simulink model "Copy_of_Corneto_flight_program_control"  (R2021a)
settings: Solver=FixedStepAuto  StartTime=0.0  StopTime=inf  RelTol=1e-3
values from neighbouring files (symbols this model uses):
  den_lpf_d = den_lpf20    [Mainframe_init.m]    (also in load_autopilot.m)
  num_lpf_d = num_lpf20    [Mainframe_init.m]    (also in load_autopilot.m)
undefined symbols (not defined in the file or in its folder): Autopilot, AUX, dev, DiscIntNeverNeededParam, Flight_Logic, HIL_Data, Main, pwm_output0, pwm_output1, severity, text, x, y, z
libraries: simulink_extras x24, simulink x22, px4uORBlib x10, px4lib x10, px4Sensorslib x6, dspstat3 x2, sharedtransform x2
(part 2 of 3)

== system Copy_of_Corneto_flight_program_control/PixBlock2/Flight Logic/Subsystem4/Servo Commands2 ==
  Fin Cmd : Inport
  Recovery : Inport  Port=2
  Bus Selector : BusSelector  OutputSignals=signal1,signal2,signal3,signal4
  Cast To Double{1..5} (5 alike) : DataTypeConversion  OutDataTypeStr=uint16
  One4 : Constant  Value=0  OutDataTypeStr=boolean
  One5 : Constant  Value=2000  OutDataTypeStr=Inherit: Inherit via back propagation
  One6 : Constant  Value=1000  OutDataTypeStr=Inherit: Inherit via back propagation
  One7 : Constant  OutDataTypeStr=boolean
  PX4 PWM Output1 : px4lib/PX4 PWM Output  pwmDevice=Main (/dev/pwm_output0)  pwmChannel1_=on  pwmChannel2_=on  pwmChannel3_=on  pwmChannel4_=on  pwmChannel5_=on  pwmChannel6_=off  pwmChannel7_=off  pwmChannel8_=off  forceTerminateFailsafe=off  outputErrorStatus=off
      settings: SourceProductBaseCode=PX4AUTOPILOTS
  Switch : Switch  Criteria=u2 > Threshold
  Pwm : Outport
  wires:
  Bus Selector/4 -> Cast To Double1/1  "<signal4>"
  One4/1 -> PX4 PWM Output1/2
  Bus Selector/3 -> Cast To Double2/1  "<signal3>"
  Bus Selector/2 -> Cast To Double3/1  "<signal2>"
  Bus Selector/1 -> Cast To Double5/1  "<signal1>"
  Cast To Double4/1 -> PX4 PWM Output1/7
  Recovery/1 -> Switch/2
  One5/1 -> Switch/1
  One6/1 -> Switch/3
  Switch/1 -> Cast To Double4/1
  One7/1 -> PX4 PWM Output1/1
  Fin Cmd/1 -> Pwm/1, Bus Selector/1
  Cast To Double1/1 -> PX4 PWM Output1/6
  Cast To Double2/1 -> PX4 PWM Output1/5
  Cast To Double3/1 -> PX4 PWM Output1/4
  Cast To Double5/1 -> PX4 PWM Output1/3

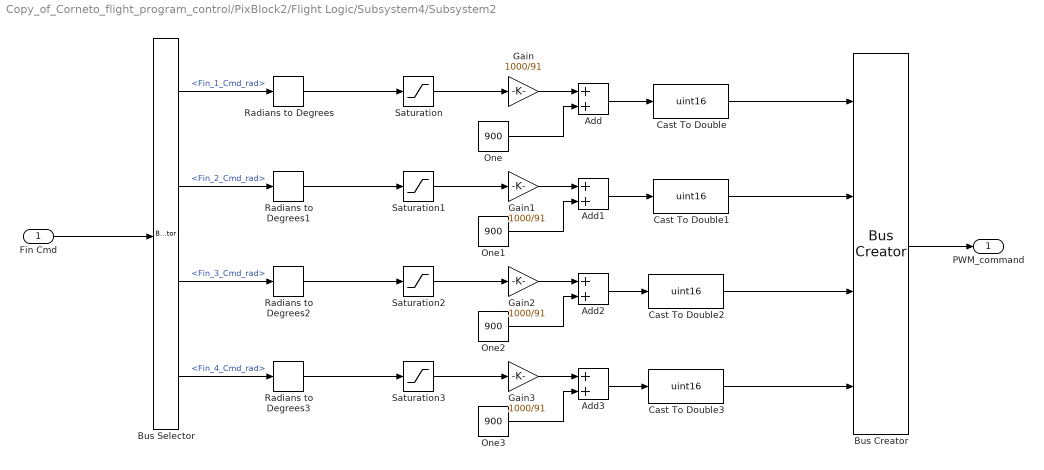
== system Copy_of_Corneto_flight_program_control/PixBlock2/Flight Logic/Subsystem4/Subsystem2 ==
  Fin Cmd : Inport
  Add{,1..3} (4 alike) : Sum
  Bus Selector : BusSelector  OutputSignals=Fin_1_Cmd_rad,Fin_2_Cmd_rad,Fin_3_Cmd_rad,Fin_4_Cmd_rad
  Bus Creator : BusCreator  Inputs=4
  Cast To Double{,1..3} (4 alike) : DataTypeConversion  OutDataTypeStr=uint16
  Gain{,1..3} (4 alike) : Gain  Gain=1000/91
  One{,1..3} (4 alike) : Constant  Value=900  OutDataTypeStr=Inherit: Inherit via back propagation
  Radians to Degrees{,1..3} (4 alike) : simulink_extras/Transformations/Radians to Degrees
  Saturation{,1..3} (4 alike) : Saturate  UpperLimit=20  LowerLimit=-20
  PWM_command : Outport
  wires:
  One2/1 -> Add2/2
  Add2/1 -> Cast To Double2/1
  Radians to Degrees2/1 -> Saturation2/1
  Cast To Double2/1 -> Bus Creator/3
  Gain/1 -> Add/1
  Bus Selector/1 -> Radians to Degrees/1  "<Fin_1_Cmd_rad>"
  Fin Cmd/1 -> Bus Selector/1
  Saturation/1 -> Gain/1
  Bus Selector/2 -> Radians to Degrees1/1  "<Fin_2_Cmd_rad>"
  Radians to Degrees/1 -> Saturation/1
  Saturation3/1 -> Gain3/1
  Cast To Double/1 -> Bus Creator/1
  Add3/1 -> Cast To Double3/1
  Gain1/1 -> Add1/1
  Saturation1/1 -> Gain1/1
  Radians to Degrees1/1 -> Saturation1/1
  Cast To Double3/1 -> Bus Creator/4
  Radians to Degrees3/1 -> Saturation3/1
  Gain2/1 -> Add2/1
  Cast To Double1/1 -> Bus Creator/2
  Bus Selector/3 -> Radians to Degrees2/1  "<Fin_3_Cmd_rad>"
  One1/1 -> Add1/2
  Bus Selector/4 -> Radians to Degrees3/1  "<Fin_4_Cmd_rad>"
  Add/1 -> Cast To Double/1
  One3/1 -> Add3/2
  Add1/1 -> Cast To Double1/1
  Gain3/1 -> Add3/1
  Saturation2/1 -> Gain2/1
  One/1 -> Add/2
  Bus Creator/1 -> PWM_command/1

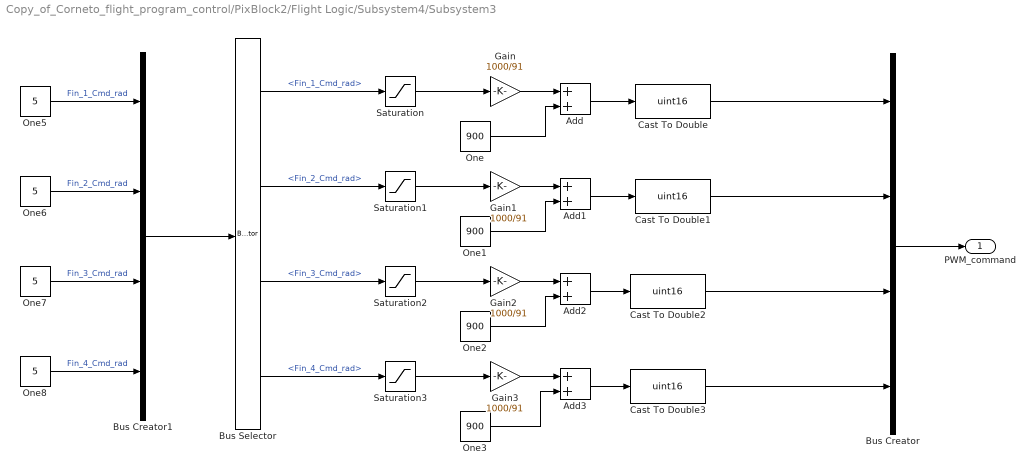
== system Copy_of_Corneto_flight_program_control/PixBlock2/Flight Logic/Subsystem4/Subsystem3 ==
  Add{,1..3} (4 alike) : Sum
  Bus Creator1 : BusCreator  Inputs=4
  Bus Selector : BusSelector  OutputSignals=Fin_1_Cmd_rad,Fin_2_Cmd_rad,Fin_3_Cmd_rad,Fin_4_Cmd_rad
  Bus Creator : BusCreator  Inputs=4
  Cast To Double{,1..3} (4 alike) : DataTypeConversion  OutDataTypeStr=uint16
  Gain{,1..3} (4 alike) : Gain  Gain=1000/91
  One{,1..3} (4 alike) : Constant  Value=900  OutDataTypeStr=Inherit: Inherit via back propagation
  One{5..8} (4 alike) : Constant  Value=5  OutDataTypeStr=Inherit: Inherit via back propagation
  Saturation{,1..3} (4 alike) : Saturate  UpperLimit=20  LowerLimit=-20
  PWM_command : Outport
  wires:
  One2/1 -> Add2/2
  Add2/1 -> Cast To Double2/1
  Cast To Double2/1 -> Bus Creator/3
  Gain/1 -> Add/1
  Bus Selector/1 -> Saturation/1  "<Fin_1_Cmd_rad>"
  Bus Creator1/1 -> Bus Selector/1
  Saturation/1 -> Gain/1
  Bus Selector/2 -> Saturation1/1  "<Fin_2_Cmd_rad>"
  Saturation3/1 -> Gain3/1
  Cast To Double/1 -> Bus Creator/1
  Add3/1 -> Cast To Double3/1
  Gain1/1 -> Add1/1
  Saturation1/1 -> Gain1/1
  Cast To Double3/1 -> Bus Creator/4
  Gain2/1 -> Add2/1
  Cast To Double1/1 -> Bus Creator/2
  Bus Selector/3 -> Saturation2/1  "<Fin_3_Cmd_rad>"
  One1/1 -> Add1/2
  Bus Selector/4 -> Saturation3/1  "<Fin_4_Cmd_rad>"
  Add/1 -> Cast To Double/1
  One3/1 -> Add3/2
  Add1/1 -> Cast To Double1/1
  Gain3/1 -> Add3/1
  Saturation2/1 -> Gain2/1
  One/1 -> Add/2
  Bus Creator/1 -> PWM_command/1
  One5/1 -> Bus Creator1/1  "Fin_1_Cmd_rad"
  One8/1 -> Bus Creator1/4  "Fin_4_Cmd_rad"
  One6/1 -> Bus Creator1/2  "Fin_2_Cmd_rad"
  One7/1 -> Bus Creator1/3  "Fin_3_Cmd_rad"

== system Copy_of_Corneto_flight_program_control/Subsystem/PixBlock2/Emulated Pixhawk/Autopilot ==
  Phi_cmd : Inport
  P_rms : Inport  Port=2
  Alt : Inport  Port=3
  Velocity : Inport  Port=4
  Phi : Inport  Port=5
  Reset_Integrators : Inport  Port=6
  Bus Creator3 : BusCreator  Inputs=3
  Discrete Transfer Fcn : DiscreteTransferFcn  Numerator=[num_lpf_d]  Denominator=[den_lpf_d]
  Phi_Control : Subsystem
  Zero : Constant  Value=0  OutDataTypeStr=Inherit: Inherit via back propagation
  Attitude_Commands : Outport  VectorParamsAs1DForOutWhenUnconnected=off
  P_filter : Outport  Port=2  VectorParamsAs1DForOutWhenUnconnected=off
  wires:
  P_rms/1 -> Discrete Transfer Fcn/1
  Velocity/1 -> Phi_Control/5(V_mps)
  Zero/1 -> [Delta_Cmd_Psi], [Delta_Cmd_Theta]
  [Delta_Cmd_Phi] -> Bus Creator3/1  "Phi_Cmd_rad"
  [Delta_Cmd_Theta] -> Bus Creator3/2  "Theta_Cmd_rad"
  Bus Creator3/1 -> Attitude_Commands/1
  [Delta_Cmd_Psi] -> Bus Creator3/3  "Psi_Cmd_rad"
  Alt/1 -> Phi_Control/6(h_m)
  Phi_Control/1(dela_cmd_rad) -> [Delta_Cmd_Phi]  "Phi_Cmd_rad"
  Discrete Transfer Fcn/1 -> P_filter/1, Phi_Control/3(p_rps)
  Phi/1 -> Phi_Control/2(phi_rad)
  Phi_cmd/1 -> Phi_Control/1(phi_cmd_rad)
  Reset_Integrators/1 -> Phi_Control/4(Reset Integrators)

== system Copy_of_Corneto_flight_program_control/Subsystem/PixBlock2/Emulated Pixhawk/Fin Allocation ==
  Attitude Cmd : Inport
  Bus Creator : BusCreator  Inputs=4
  Bus Selector : BusSelector  OutputSignals=Phi_Cmd_rad,Theta_Cmd_rad,Psi_Cmd_rad
  Demux : Demux
  Vector Concatenate1 : Concatenate  NumInputs=3
  control_allocation : Subsystem
  Fin Cmd : Outport  VectorParamsAs1DForOutWhenUnconnected=off
  wires:
  Demux/4 -> Bus Creator/4  "Fin_4_Cmd_rad"
  control_allocation/1(siB_cmd) -> Demux/1
  Bus Selector/3 -> Vector Concatenate1/3  "<Psi_Cmd_rad>"
  Vector Concatenate1/1 -> control_allocation/1(fin_cmd)  "fin_cmd"
  Bus Selector/1 -> Vector Concatenate1/1  "<Phi_Cmd_rad>"
  Demux/3 -> Bus Creator/3  "Fin_3_Cmd_rad"
  Bus Selector/2 -> Vector Concatenate1/2  "<Theta_Cmd_rad>"
  Demux/1 -> Bus Creator/1  "Fin_1_Cmd_rad"
  Bus Creator/1 -> Fin Cmd/1
  Attitude Cmd/1 -> Bus Selector/1
  Demux/2 -> Bus Creator/2  "Fin_2_Cmd_rad"

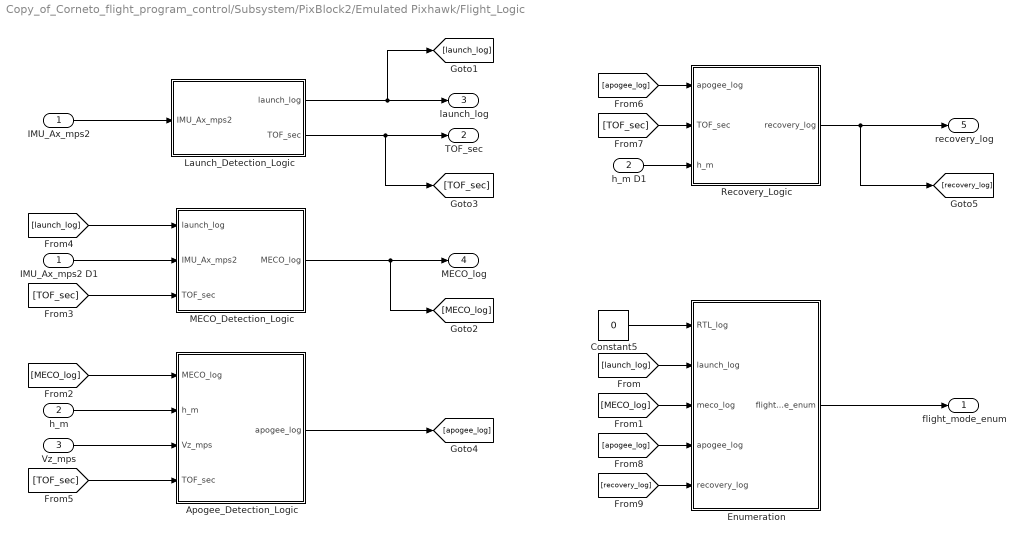
== system Copy_of_Corneto_flight_program_control/Subsystem/PixBlock2/Emulated Pixhawk/Flight_Logic ==
  IMU_Ax_mps2 : Inport
  h_m : Inport  Port=2
  Vz_mps : Inport  Port=3
  Apogee_Detection_Logic : Subsystem
  Constant5 : Constant  Value=0
  Enumeration : Subsystem
  IMU_Ax_mps2 D1 : InportShadow
  Launch_Detection_Logic : Subsystem
  MECO_Detection_Logic : Subsystem
  Recovery_Logic : Subsystem
  h_m D1 : InportShadow  Port=2
  flight_mode_enum : Outport
  TOF_sec : Outport  Port=2
  launch_log : Outport  Port=3
  MECO_log : Outport  Port=4
  recovery_log : Outport  Port=5
  wires:
  Enumeration/1(flight_mode_enum) -> flight_mode_enum/1
  [launch_log] -> Enumeration/2(launch_log)
  [MECO_log] -> Enumeration/3(meco_log)
  IMU_Ax_mps2/1 -> Launch_Detection_Logic/1(IMU_Ax_mps2)
  IMU_Ax_mps2 D1/1 -> MECO_Detection_Logic/2(IMU_Ax_mps2)
  Launch_Detection_Logic/1(launch_log) -> [launch_log], launch_log/1
  Launch_Detection_Logic/2(TOF_sec) -> [TOF_sec], TOF_sec/1
  [launch_log] -> MECO_Detection_Logic/1(launch_log)
  MECO_Detection_Logic/1(MECO_log) -> [MECO_log], MECO_log/1
  [MECO_log] -> Apogee_Detection_Logic/1(MECO_log)
  h_m/1 -> Apogee_Detection_Logic/2(h_m)
  Vz_mps/1 -> Apogee_Detection_Logic/3(Vz_mps)
  Apogee_Detection_Logic/1(apogee_log) -> [apogee_log]
  [TOF_sec] -> MECO_Detection_Logic/3(TOF_sec)
  [TOF_sec] -> Apogee_Detection_Logic/4(TOF_sec)
  Constant5/1 -> Enumeration/1(RTL_log)
  [apogee_log] -> Recovery_Logic/1(apogee_log)
  [TOF_sec] -> Recovery_Logic/2(TOF_sec)
  h_m D1/1 -> Recovery_Logic/3(h_m)
  Recovery_Logic/1(recovery_log) -> [recovery_log], recovery_log/1
  [apogee_log] -> Enumeration/4(apogee_log)
  [recovery_log] -> Enumeration/5(recovery_log)

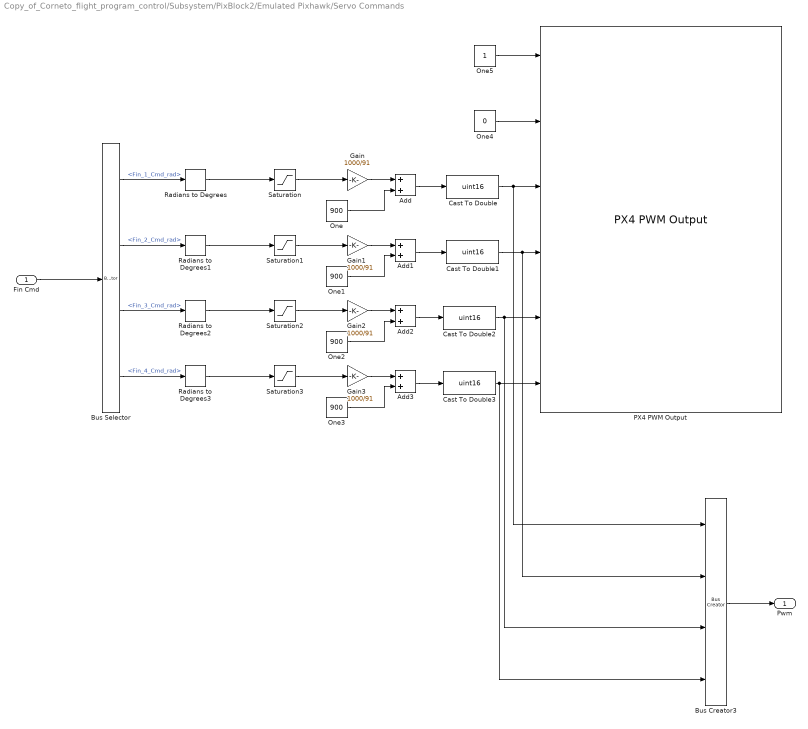
== system Copy_of_Corneto_flight_program_control/Subsystem/PixBlock2/Emulated Pixhawk/Servo Commands ==
  Fin Cmd : Inport
  Add{,1..3} (4 alike) : Sum
  Bus Creator3 : BusCreator  Inputs=4
  Bus Selector : BusSelector  OutputSignals=Fin_1_Cmd_rad,Fin_2_Cmd_rad,Fin_3_Cmd_rad,Fin_4_Cmd_rad
  Cast To Double{,1..3} (4 alike) : DataTypeConversion  OutDataTypeStr=uint16
  Gain{,1..3} (4 alike) : Gain  Gain=1000/91
  One{,1..3} (4 alike) : Constant  Value=900  OutDataTypeStr=Inherit: Inherit via back propagation
  One4 : Constant  Value=0  OutDataTypeStr=boolean  SampleTime=-1
  One5 : Constant  OutDataTypeStr=boolean  SampleTime=-1
  PX4 PWM Output : px4lib/PX4 PWM Output  pwmDevice=AUX (/dev/pwm_output1)  pwmChannel1_=on  pwmChannel2_=on  pwmChannel3_=on  pwmChannel4_=on  pwmChannel5_=off  pwmChannel6_=off  pwmChannel7_=off  pwmChannel8_=off  forceTerminateFailsafe=off  outputErrorStatus=off
      settings: SourceProductBaseCode=PX4AUTOPILOTS
  Radians to Degrees{,1..3} (4 alike) : simulink_extras/Transformations/Radians to Degrees
  Saturation{,1..3} (4 alike) : Saturate  UpperLimit=20  LowerLimit=-20
  Pwm : Outport
  wires:
  Saturation2/1 -> Gain2/1
  One4/1 -> PX4 PWM Output/2
  One/1 -> Add/2
  One2/1 -> Add2/2
  Add1/1 -> Cast To Double1/1
  Gain2/1 -> Add2/1
  Radians to Degrees1/1 -> Saturation1/1
  Add2/1 -> Cast To Double2/1
  Fin Cmd/1 -> Bus Selector/1
  Bus Selector/2 -> Radians to Degrees1/1  "<Fin_2_Cmd_rad>"
  Gain/1 -> Add/1
  Bus Selector/4 -> Radians to Degrees3/1  "<Fin_4_Cmd_rad>"
  One3/1 -> Add3/2
  Saturation/1 -> Gain/1
  Gain1/1 -> Add1/1
  Saturation3/1 -> Gain3/1
  Gain3/1 -> Add3/1
  Radians to Degrees3/1 -> Saturation3/1
  Bus Selector/1 -> Radians to Degrees/1  "<Fin_1_Cmd_rad>"
  Bus Selector/3 -> Radians to Degrees2/1  "<Fin_3_Cmd_rad>"
  Saturation1/1 -> Gain1/1
  Add3/1 -> Cast To Double3/1
  Radians to Degrees2/1 -> Saturation2/1
  Radians to Degrees/1 -> Saturation/1
  One1/1 -> Add1/2
  Add/1 -> Cast To Double/1
  Bus Creator3/1 -> Pwm/1
  Cast To Double/1 -> PX4 PWM Output/3, Bus Creator3/1
  Cast To Double1/1 -> PX4 PWM Output/4, Bus Creator3/2
  Cast To Double2/1 -> PX4 PWM Output/5, Bus Creator3/3
  Cast To Double3/1 -> PX4 PWM Output/6, Bus Creator3/4
  One5/1 -> PX4 PWM Output/1

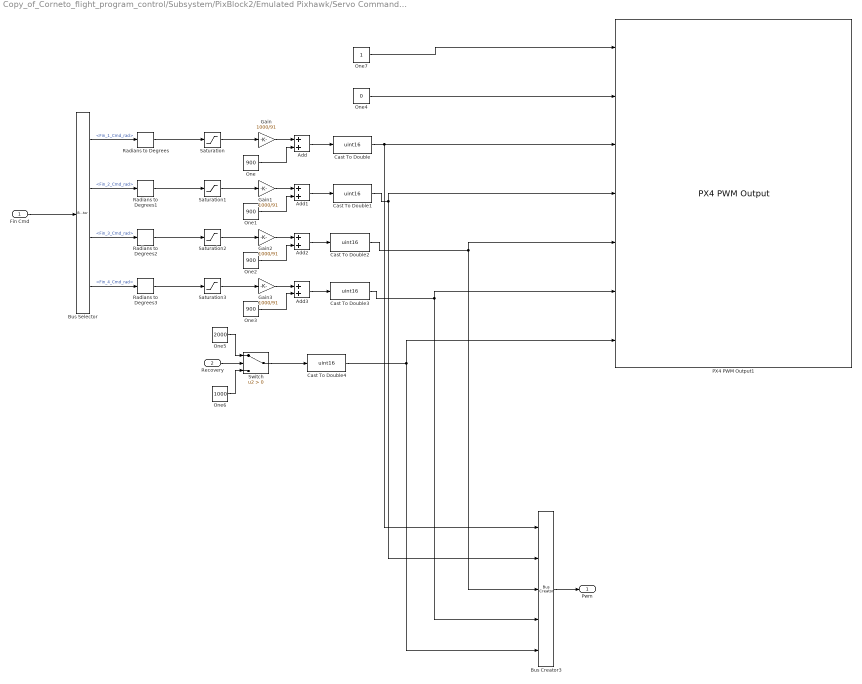
== system Copy_of_Corneto_flight_program_control/Subsystem/PixBlock2/Emulated Pixhawk/Servo Commands1 ==
  Fin Cmd : Inport
  Recovery : Inport  Port=2
  Add{,1..3} (4 alike) : Sum
  Bus Creator3 : BusCreator  Inputs=5
  Bus Selector : BusSelector  OutputSignals=Fin_1_Cmd_rad,Fin_2_Cmd_rad,Fin_3_Cmd_rad,Fin_4_Cmd_rad
  Cast To Double{,1..4} (5 alike) : DataTypeConversion  OutDataTypeStr=uint16
  Gain{,1..3} (4 alike) : Gain  Gain=1000/91
  One{,1..3} (4 alike) : Constant  Value=900  OutDataTypeStr=Inherit: Inherit via back propagation
  One4 : Constant  Value=0  OutDataTypeStr=boolean
  One5 : Constant  Value=2000  OutDataTypeStr=Inherit: Inherit via back propagation
  One6 : Constant  Value=1000  OutDataTypeStr=Inherit: Inherit via back propagation
  One7 : Constant  OutDataTypeStr=boolean
  PX4 PWM Output1 : px4lib/PX4 PWM Output  pwmDevice=Main (/dev/pwm_output0)  pwmChannel1_=on  pwmChannel2_=on  pwmChannel3_=on  pwmChannel4_=on  pwmChannel5_=on  pwmChannel6_=off  pwmChannel7_=off  pwmChannel8_=off  forceTerminateFailsafe=off  outputErrorStatus=off
      settings: SourceProductBaseCode=PX4AUTOPILOTS
  Radians to Degrees{,1..3} (4 alike) : simulink_extras/Transformations/Radians to Degrees
  Saturation{,1..3} (4 alike) : Saturate  UpperLimit=20  LowerLimit=-20
  Switch : Switch  Criteria=u2 > Threshold
  Pwm : Outport
  wires:
  Saturation2/1 -> Gain2/1
  Cast To Double3/1 -> Bus Creator3/4, PX4 PWM Output1/6
  One4/1 -> PX4 PWM Output1/2
  One/1 -> Add/2
  One2/1 -> Add2/2
  Add1/1 -> Cast To Double1/1
  Gain2/1 -> Add2/1
  Radians to Degrees1/1 -> Saturation1/1
  Cast To Double2/1 -> Bus Creator3/3, PX4 PWM Output1/5
  Add2/1 -> Cast To Double2/1
  Fin Cmd/1 -> Bus Selector/1
  Cast To Double1/1 -> Bus Creator3/2, PX4 PWM Output1/4
  Bus Selector/2 -> Radians to Degrees1/1  "<Fin_2_Cmd_rad>"
  Gain/1 -> Add/1
  Bus Selector/4 -> Radians to Degrees3/1  "<Fin_4_Cmd_rad>"
  One3/1 -> Add3/2
  Saturation/1 -> Gain/1
  Gain1/1 -> Add1/1
  Saturation3/1 -> Gain3/1
  Gain3/1 -> Add3/1
  Radians to Degrees3/1 -> Saturation3/1
  Bus Selector/1 -> Radians to Degrees/1  "<Fin_1_Cmd_rad>"
  Bus Selector/3 -> Radians to Degrees2/1  "<Fin_3_Cmd_rad>"
  Saturation1/1 -> Gain1/1
  Cast To Double/1 -> Bus Creator3/1, PX4 PWM Output1/3
  Add3/1 -> Cast To Double3/1
  Radians to Degrees2/1 -> Saturation2/1
  Radians to Degrees/1 -> Saturation/1
  One1/1 -> Add1/2
  Add/1 -> Cast To Double/1
  Cast To Double4/1 -> Bus Creator3/5, PX4 PWM Output1/7
  Recovery/1 -> Switch/2
  One5/1 -> Switch/1
  One6/1 -> Switch/3
  Switch/1 -> Cast To Double4/1
  One7/1 -> PX4 PWM Output1/1
  Bus Creator3/1 -> Pwm/1

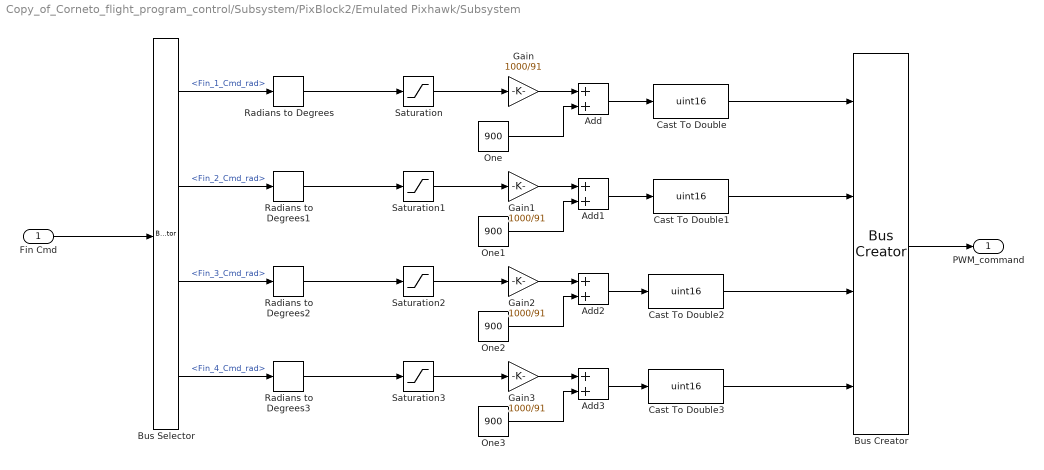
== system Copy_of_Corneto_flight_program_control/Subsystem/PixBlock2/Emulated Pixhawk/Subsystem ==
  Fin Cmd : Inport
  Add{,1..3} (4 alike) : Sum
  Bus Selector : BusSelector  OutputSignals=Fin_1_Cmd_rad,Fin_2_Cmd_rad,Fin_3_Cmd_rad,Fin_4_Cmd_rad
  Bus Creator : BusCreator  Inputs=4
  Cast To Double{,1..3} (4 alike) : DataTypeConversion  OutDataTypeStr=uint16
  Gain{,1..3} (4 alike) : Gain  Gain=1000/91
  One{,1..3} (4 alike) : Constant  Value=900  OutDataTypeStr=Inherit: Inherit via back propagation
  Radians to Degrees{,1..3} (4 alike) : simulink_extras/Transformations/Radians to Degrees
  Saturation{,1..3} (4 alike) : Saturate  UpperLimit=20  LowerLimit=-20
  PWM_command : Outport
  wires:
  One2/1 -> Add2/2
  Add2/1 -> Cast To Double2/1
  Radians to Degrees2/1 -> Saturation2/1
  Cast To Double2/1 -> Bus Creator/3
  Gain/1 -> Add/1
  Bus Selector/1 -> Radians to Degrees/1  "<Fin_1_Cmd_rad>"
  Fin Cmd/1 -> Bus Selector/1
  Saturation/1 -> Gain/1
  Bus Selector/2 -> Radians to Degrees1/1  "<Fin_2_Cmd_rad>"
  Radians to Degrees/1 -> Saturation/1
  Saturation3/1 -> Gain3/1
  Cast To Double/1 -> Bus Creator/1
  Add3/1 -> Cast To Double3/1
  Gain1/1 -> Add1/1
  Saturation1/1 -> Gain1/1
  Radians to Degrees1/1 -> Saturation1/1
  Cast To Double3/1 -> Bus Creator/4
  Radians to Degrees3/1 -> Saturation3/1
  Gain2/1 -> Add2/1
  Cast To Double1/1 -> Bus Creator/2
  Bus Selector/3 -> Radians to Degrees2/1  "<Fin_3_Cmd_rad>"
  One1/1 -> Add1/2
  Bus Selector/4 -> Radians to Degrees3/1  "<Fin_4_Cmd_rad>"
  Add/1 -> Cast To Double/1
  One3/1 -> Add3/2
  Add1/1 -> Cast To Double1/1
  Gain3/1 -> Add3/1
  Saturation2/1 -> Gain2/1
  One/1 -> Add/2
  Bus Creator/1 -> PWM_command/1

== system Copy_of_Corneto_flight_program_control/Subsystem/PixBlock2/Emulated Pixhawk/Subsystem1 ==
  Add{,1..3} (4 alike) : Sum
  Bus Creator1 : BusCreator  Inputs=4
  Bus Selector : BusSelector  OutputSignals=Fin_1_Cmd_rad,Fin_2_Cmd_rad,Fin_3_Cmd_rad,Fin_4_Cmd_rad
  Bus Creator : BusCreator  Inputs=4
  Cast To Double{,1..3} (4 alike) : DataTypeConversion  OutDataTypeStr=uint16
  Gain{,1..3} (4 alike) : Gain  Gain=1000/91
  One{,1..3} (4 alike) : Constant  Value=900  OutDataTypeStr=Inherit: Inherit via back propagation
  One{5..8} (4 alike) : Constant  Value=5  OutDataTypeStr=Inherit: Inherit via back propagation
  Saturation{,1..3} (4 alike) : Saturate  UpperLimit=20  LowerLimit=-20
  PWM_command : Outport
  wires:
  One2/1 -> Add2/2
  Add2/1 -> Cast To Double2/1
  Cast To Double2/1 -> Bus Creator/3
  Gain/1 -> Add/1
  Bus Selector/1 -> Saturation/1  "<Fin_1_Cmd_rad>"
  Bus Creator1/1 -> Bus Selector/1
  Saturation/1 -> Gain/1
  Bus Selector/2 -> Saturation1/1  "<Fin_2_Cmd_rad>"
  Saturation3/1 -> Gain3/1
  Cast To Double/1 -> Bus Creator/1
  Add3/1 -> Cast To Double3/1
  Gain1/1 -> Add1/1
  Saturation1/1 -> Gain1/1
  Cast To Double3/1 -> Bus Creator/4
  Gain2/1 -> Add2/1
  Cast To Double1/1 -> Bus Creator/2
  Bus Selector/3 -> Saturation2/1  "<Fin_3_Cmd_rad>"
  One1/1 -> Add1/2
  Bus Selector/4 -> Saturation3/1  "<Fin_4_Cmd_rad>"
  Add/1 -> Cast To Double/1
  One3/1 -> Add3/2
  Add1/1 -> Cast To Double1/1
  Gain3/1 -> Add3/1
  Saturation2/1 -> Gain2/1
  One/1 -> Add/2
  Bus Creator/1 -> PWM_command/1
  One5/1 -> Bus Creator1/1  "Fin_1_Cmd_rad"
  One8/1 -> Bus Creator1/4  "Fin_4_Cmd_rad"
  One6/1 -> Bus Creator1/2  "Fin_2_Cmd_rad"
  One7/1 -> Bus Creator1/3  "Fin_3_Cmd_rad"

== system Copy_of_Corneto_flight_program_control/PixBlock2/Flight Logic/Autopilot/Phi_Control/Gain_Lookup ==
  V_mps : Inport
  h_m : Inport  Port=2
  1-D Lookup Table1 : Lookup_n-D  BreakpointsForDimension1=Autopilot.Ay.h_bkpts_m  BreakpointsForDimension2=Autopilot.Ay.V_bkpts_mps  Table=Autopilot.Ay.Kp_r_vec  ExtrapMethod=Clip  UseLastTableValue=on  InternalRulePriority=Speed  RndMeth=Simplest  InputSameDT=on
      settings: InputPortMap=u0,u1
      settings: AttributesFormatString=|
      | %<Table>
      | %<BreakpointsForDimension1>
      | %<BreakpointsForDimension2>
  1-D Lookup Table2 : Lookup_n-D  BreakpointsForDimension1=Autopilot.Ay.h_bkpts_m  BreakpointsForDimension2=Autopilot.Ay.V_bkpts_mps  Table=Autopilot.Ay.Kp_ay_vec  ExtrapMethod=Clip  UseLastTableValue=on  InternalRulePriority=Speed  RndMeth=Simplest  InputSameDT=on
      settings: InputPortMap=u0,u1
      settings: AttributesFormatString=|
      | %<Table>
      | %<BreakpointsForDimension1>
      | %<BreakpointsForDimension2>
  1-D Lookup Table3 : Lookup_n-D  BreakpointsForDimension1=Autopilot.Phi.h_bkpts_m  BreakpointsForDimension2=Autopilot.Phi.V_bkpts_mps  Table=Autopilot.Phi.Kp_p_vec  ExtrapMethod=Clip  UseLastTableValue=on  InternalRulePriority=Speed  RndMeth=Simplest  InputSameDT=on
      settings: InputPortMap=u0,u1
      settings: AttributesFormatString=|
      | %<Table>
      | %<BreakpointsForDimension1>
      | %<BreakpointsForDimension2>
  1-D Lookup Table4 : Lookup_n-D  BreakpointsForDimension1=Autopilot.Phi.h_bkpts_m  BreakpointsForDimension2=Autopilot.Phi.V_bkpts_mps  Table=Autopilot.Phi.Ki_phi_vec  ExtrapMethod=Clip  UseLastTableValue=on  InternalRulePriority=Speed  RndMeth=Simplest  InputSameDT=on
      settings: InputPortMap=u0,u1
      settings: AttributesFormatString=|
      | %<Table>
      | %<BreakpointsForDimension1>
      | %<BreakpointsForDimension2>
  1-D Lookup Table5 : Lookup_n-D  BreakpointsForDimension1=Autopilot.Phi.h_bkpts_m  BreakpointsForDimension2=Autopilot.Phi.V_bkpts_mps  Table=Autopilot.Phi.Kp_phi_vec  ExtrapMethod=Clip  UseLastTableValue=on  InternalRulePriority=Speed  RndMeth=Simplest  InputSameDT=on
      settings: InputPortMap=u0,u1
      settings: AttributesFormatString=|
      | %<Table>
      | %<BreakpointsForDimension1>
      | %<BreakpointsForDimension2>
  1-D Lookup Table6 : Lookup_n-D  BreakpointsForDimension1=Autopilot.Ay.h_bkpts_m  BreakpointsForDimension2=Autopilot.Ay.V_bkpts_mps  Table=Autopilot.Ay.Ki_ay_vec  ExtrapMethod=Clip  UseLastTableValue=on  InternalRulePriority=Speed  RndMeth=Simplest  InputSameDT=on
      settings: InputPortMap=u0,u1
      settings: AttributesFormatString=|
      | %<Table>
      | %<BreakpointsForDimension1>
      | %<BreakpointsForDimension2>
  Bus Creator1 : BusCreator  Inputs=6
  V_mps D{1..5} (5 alike) : InportShadow
  h_m D{1..5} (5 alike) : InportShadow  Port=2
  Gains : Outport
  wires:
  h_m/1 -> 1-D Lookup Table3/1
  Bus Creator1/1 -> Gains/1
  1-D Lookup Table5/1 -> Bus Creator1/3  "Kp_phi"
  1-D Lookup Table4/1 -> Bus Creator1/2  "Ki_phi"
  1-D Lookup Table3/1 -> Bus Creator1/1  "Kp_p"
  V_mps/1 -> 1-D Lookup Table3/2
  h_m D1/1 -> 1-D Lookup Table4/1
  V_mps D1/1 -> 1-D Lookup Table4/2
  h_m D2/1 -> 1-D Lookup Table5/1
  V_mps D2/1 -> 1-D Lookup Table5/2
  1-D Lookup Table2/1 -> Bus Creator1/6  "Kp_ay"
  1-D Lookup Table6/1 -> Bus Creator1/5  "Ki_ay"
  1-D Lookup Table1/1 -> Bus Creator1/4  "Kp_r"
  h_m D3/1 -> 1-D Lookup Table1/1
  V_mps D3/1 -> 1-D Lookup Table1/2
  h_m D4/1 -> 1-D Lookup Table6/1
  V_mps D4/1 -> 1-D Lookup Table6/2
  h_m D5/1 -> 1-D Lookup Table2/1
  V_mps D5/1 -> 1-D Lookup Table2/2

== system Copy_of_Corneto_flight_program_control/PixBlock2/Flight Logic/Flight_Logic/Apogee_Detection_Logic/Enable_Timer_Logic ==
  enable_timer : Inport
  Constant : Constant
  Constant1 : Constant  Value=0
  Discrete-Time Integrator : DiscreteIntegrator  ExternalReset=level  InitialConditionSource=external  SampleTime=-1  ICPrevOutput=DiscIntNeverNeededParam  ICPrevScaledInput=DiscIntNeverNeededParam
  NOT : Logic  Operator=NOT  AllPortsSameDT=off  OutDataTypeStr=boolean
  timer : Outport
  wires:
  NOT/1 -> Discrete-Time Integrator/2
  Discrete-Time Integrator/1 -> timer/1  "apogee_detect_timer_sec"
  Constant1/1 -> Discrete-Time Integrator/3
  Constant/1 -> Discrete-Time Integrator/1
  enable_timer/1 -> NOT/1  "enable_timer"

== system Copy_of_Corneto_flight_program_control/PixBlock2/Flight Logic/Flight_Logic/Apogee_Detection_Logic/Latch_Signal ==
  signal : Inport
  Memory : Memory  InheritSampleTime=on
  Switch1 : Switch  Criteria=u2 ~= 0
      settings: AttributesFormatString=%<Criteria>
  signal_latched : Outport
  wires:
  signal/1 -> Switch1/2, Switch1/1
  Switch1/1 -> Memory/1, signal_latched/1
  Memory/1 -> Switch1/3

== system Copy_of_Corneto_flight_program_control/PixBlock2/Flight Logic/Flight_Logic/Launch_Detection_Logic/Enable_Timer_Logic ==
  accel_threshold_log : Inport
  launch_latched : Inport  Port=2
  AND : Logic  Operator=OR  AllPortsSameDT=off  OutDataTypeStr=boolean
  Constant : Constant
  Constant1 : Constant  Value=0
  Discrete-Time Integrator : DiscreteIntegrator  ExternalReset=level  InitialConditionSource=external  SampleTime=-1  ICPrevOutput=DiscIntNeverNeededParam  ICPrevScaledInput=DiscIntNeverNeededParam
  NOT : Logic  Operator=NOT  AllPortsSameDT=off  OutDataTypeStr=boolean
  time_since_launch : Outport
  wires:
  launch_latched/1 -> AND/2
  AND/1 -> NOT/1  "enable_timer"
  Constant/1 -> Discrete-Time Integrator/1
  Constant1/1 -> Discrete-Time Integrator/3
  Discrete-Time Integrator/1 -> time_since_launch/1  "launch_detect_timer_sec"
  accel_threshold_log/1 -> AND/1
  NOT/1 -> Discrete-Time Integrator/2

== system Copy_of_Corneto_flight_program_control/PixBlock2/Flight Logic/Flight_Logic/Launch_Detection_Logic/Latch_Signal ==
  signal : Inport
  Memory : Memory  InheritSampleTime=on  LinearizeAsDelay=on
  Switch1 : Switch  Criteria=u2 ~= 0
      settings: AttributesFormatString=%<Criteria>
  signal_latched : Outport
  wires:
  Memory/1 -> Switch1/3
  Switch1/1 -> signal_latched/1, Memory/1
  signal/1 -> Switch1/1, Switch1/2

== system Copy_of_Corneto_flight_program_control/PixBlock2/Flight Logic/Flight_Logic/MECO_Detection_Logic/Enable_Timer_Logic ==
  enable_timer : Inport
  Constant : Constant
  Constant1 : Constant  Value=0
  Discrete-Time Integrator : DiscreteIntegrator  ExternalReset=level  InitialConditionSource=external  SampleTime=-1  ICPrevOutput=DiscIntNeverNeededParam  ICPrevScaledInput=DiscIntNeverNeededParam
  NOT : Logic  Operator=NOT  AllPortsSameDT=off  OutDataTypeStr=boolean
  timer : Outport
  wires:
  enable_timer/1 -> NOT/1  "enable_timer"
  Constant/1 -> Discrete-Time Integrator/1
  Constant1/1 -> Discrete-Time Integrator/3
  Discrete-Time Integrator/1 -> timer/1  "MECO_detect_timer_sec"
  NOT/1 -> Discrete-Time Integrator/2

== system Copy_of_Corneto_flight_program_control/PixBlock2/Flight Logic/Flight_Logic/MECO_Detection_Logic/Latch_Signal ==
  signal : Inport
  Memory : Memory  InheritSampleTime=on
  Switch1 : Switch  Criteria=u2 ~= 0
      settings: AttributesFormatString=%<Criteria>
  signal_latched : Outport
  wires:
  Memory/1 -> Switch1/3
  Switch1/1 -> signal_latched/1, Memory/1
  signal/1 -> Switch1/1, Switch1/2

== system Copy_of_Corneto_flight_program_control/PixBlock2/Flight Logic/Flight_Logic/Recovery_Logic/Enable_Timer_Logic ==
  enable_timer : Inport
  Constant : Constant
  Constant1 : Constant  Value=0
  Discrete-Time Integrator : DiscreteIntegrator  ExternalReset=level  InitialConditionSource=external  SampleTime=-1  ICPrevOutput=DiscIntNeverNeededParam  ICPrevScaledInput=DiscIntNeverNeededParam
  NOT : Logic  Operator=NOT  AllPortsSameDT=off  OutDataTypeStr=boolean
  timer : Outport
  wires:
  NOT/1 -> Discrete-Time Integrator/2
  Discrete-Time Integrator/1 -> timer/1  "recovery_detect_timer_sec"
  Constant1/1 -> Discrete-Time Integrator/3
  Constant/1 -> Discrete-Time Integrator/1
  enable_timer/1 -> NOT/1  "enable_timer"

== system Copy_of_Corneto_flight_program_control/PixBlock2/Flight Logic/Flight_Logic/Recovery_Logic/Latch_Signal ==
  signal : Inport
  Memory : Memory  InheritSampleTime=on
  Switch1 : Switch  Criteria=u2 ~= 0
      settings: AttributesFormatString=%<Criteria>
  signal_latched : Outport
  wires:
  signal/1 -> Switch1/2, Switch1/1
  Switch1/1 -> Memory/1, signal_latched/1
  Memory/1 -> Switch1/3

== system Copy_of_Corneto_flight_program_control/Subsystem/PixBlock2/Emulated Pixhawk/Autopilot/Phi_Control ==
  phi_cmd_rad : Inport
  phi_rad : Inport  Port=2
  p_rps : Inport  Port=3
  Reset Integrators : Inport  Port=4
  V_mps : Inport  Port=5
  h_m : Inport  Port=6
  Bus Selector : BusSelector  OutputSignals=Kp_p,Ki_phi,Kp_phi,Kp_r,Ki_ay,Kp_ay
  Constant : Constant  Value=0  OutDataTypeStr=single  SampleTime=-1
  Discrete-Time Integrator : DiscreteIntegrator  ExternalReset=level  InitialConditionSource=external  SampleTime=-1  OutDataTypeStr=single  ICPrevOutput=DiscIntNeverNeededParam  ICPrevScaledInput=DiscIntNeverNeededParam
  Gain_Lookup : Subsystem
  Product1 : Product
  Product2 : Product
  Product3 : Product
  Sum3 : Sum  Inputs=|+-
  Sum4 : Sum  Inputs=++|
  Sum5 : Sum  Inputs=|+-
  dela_cmd_rad : Outport
  wires:
  phi_cmd_rad/1 -> Sum3/1
  Reset Integrators/1 -> Discrete-Time Integrator/2
  p_rps/1 -> Sum5/2
  phi_rad/1 -> Sum3/2
  Product2/1 -> Sum4/1
  Sum3/1 -> Product3/2, Product2/2
  Constant/1 -> Discrete-Time Integrator/3
  Sum5/1 -> Product1/2
  [Ki_phi] -> Product3/1
  Product1/1 -> dela_cmd_rad/1
  [Kp_p] -> Product1/1
  [Kp_phi] -> Product2/1
  Discrete-Time Integrator/1 -> Sum4/2  "phi_int"
  Sum4/1 -> Sum5/1
  Product3/1 -> Discrete-Time Integrator/1
  h_m/1 -> Gain_Lookup/2(h_m)
  Bus Selector/6 -> [Kp_ay]  "<Kp_ay>"
  Bus Selector/5 -> [Ki_ay]  "<Ki_ay>"
  Bus Selector/2 -> [Ki_phi]  "<Ki_phi>"
  Bus Selector/1 -> [Kp_p]  "<Kp_p>"
  V_mps/1 -> Gain_Lookup/1(V_mps)
  Bus Selector/4 -> [Kp_r]  "<Kp_r>"
  Gain_Lookup/1(Gains) -> Bus Selector/1
  Bus Selector/3 -> [Kp_phi]  "<Kp_phi>"

== system Copy_of_Corneto_flight_program_control/Subsystem/PixBlock2/Emulated Pixhawk/Fin Allocation/control_allocation ==
  fin_cmd : Inport
  Constant7 : Constant  Value=HIL_Data.FDM.Tr4r3  OutDataTypeStr=single
  Product : Product  Multiplication=Matrix(*)
  siB_cmd : Outport  VectorParamsAs1DForOutWhenUnconnected=off
  wires:
  Constant7/1 -> Product/1
  fin_cmd/1 -> Product/2
  Product/1 -> siB_cmd/1  "siB_cmd"

== system Copy_of_Corneto_flight_program_control/Subsystem/PixBlock2/Emulated Pixhawk/Flight_Logic/Apogee_Detection_Logic ==
  MECO_log : Inport
  h_m : Inport  Port=2
  Vz_mps : Inport  Port=3
  TOF_sec : Inport  Port=4
  AND : Logic  Inputs=3  AllPortsSameDT=off  OutDataTypeStr=boolean
  AND1 : Logic  Operator=OR  AllPortsSameDT=off  OutDataTypeStr=boolean
  Compare To Constant : simulink/Logic and Bit Operations/Compare To Constant  relop=>  const=0  OutDataTypeStr=boolean
  Compare To Constant1 : simulink/Logic and Bit Operations/Compare To Constant  relop=>=  const=Flight_Logic.h_apogee_timer_threshold_sec  OutDataTypeStr=boolean
      settings: AttributesFormatString=|
      | %<relop>
      | %<const>
  Compare To Constant3 : simulink/Logic and Bit Operations/Compare To Constant  relop=>=  const=Flight_Logic.apogee_timeout_TOF_sec  OutDataTypeStr=boolean
      settings: AttributesFormatString=|
      | %<relop>
      | %<const>
  Detect Decrease : simulink/Logic and Bit Operations/Detect Decrease  vinit=0.0  OutDataTypeStr=uint8
  Enable_Timer_Logic : Subsystem
  Latch_Signal : Subsystem
  Moving Average1 : dspstat3/Moving Average  Method=Sliding window  ForgettingFactorPort=off  SpecifyWindowLength=on  WindowLength=guidc_n_window  ForgettingFactor=0.9  SimulateUsing=Code generation
  apogee_log : Outport
  wires:
  AND1/1 -> apogee_log/1  "apogee_log"
  AND/1 -> Latch_Signal/1(signal)
  h_m/1 -> Moving Average1/1
  MECO_log/1 -> AND/1
  Moving Average1/1 -> Detect Decrease/1  "hBE_mf"
  Detect Decrease/1 -> Enable_Timer_Logic/1(enable_timer)  "flag_I_hBE"
  Enable_Timer_Logic/1(timer) -> Compare To Constant1/1
  Compare To Constant1/1 -> AND/2  "apogee_timer_log"
  Vz_mps/1 -> Compare To Constant/1
  Compare To Constant/1 -> AND/3  "apogee_vz_log"
  Latch_Signal/1(signal_latched) -> AND1/1  "apogee_latched"
  TOF_sec/1 -> Compare To Constant3/1
  Compare To Constant3/1 -> AND1/2  "apogee_timeout_log"

== system Copy_of_Corneto_flight_program_control/Subsystem/PixBlock2/Emulated Pixhawk/Flight_Logic/Enumeration ==
  RTL_log : Inport
  launch_log : Inport  Port=2
  meco_log : Inport  Port=3
  apogee_log : Inport  Port=4
  recovery_log : Inport  Port=5
  Constant : Constant
  Constant1 : Constant  Value=200
  Constant2 : Constant  Value=300
  Constant3 : Constant  Value=400
  Constant4 : Constant  Value=600
  Constant5 : Constant  Value=0
  Constant6 : Constant  Value=500
  Switch{,1..4} (5 alike) : Switch  Criteria=u2 ~= 0
  Terminator : Terminator
  flight_mode_enum : Outport
  wires:
  Switch/1 -> Switch1/3
  Constant3/1 -> Switch2/1
  Constant4/1 -> Switch3/1
  RTL_log/1 -> Switch/2
  Constant1/1 -> Switch/1
  Constant/1 -> Switch/3
  Switch3/1 -> flight_mode_enum/1  "flight_mode_enum"
  meco_log/1 -> Switch2/2
  launch_log/1 -> Switch1/2
  Constant2/1 -> Switch1/1
  Switch2/1 -> Switch4/3
  Switch1/1 -> Switch2/3
  Constant5/1 -> Switch4/2
  Constant6/1 -> Switch4/1
  Switch4/1 -> Switch3/3
  recovery_log/1 -> Switch3/2
  apogee_log/1 -> Terminator/1

== system Copy_of_Corneto_flight_program_control/Subsystem/PixBlock2/Emulated Pixhawk/Flight_Logic/Launch_Detection_Logic ==
  IMU_Ax_mps2 : Inport
  AND : Logic  AllPortsSameDT=off  OutDataTypeStr=boolean
  Compare To Constant : simulink/Logic and Bit Operations/Compare To Constant  relop=>=  const=Flight_Logic.Ax_launch_accel_threshold_mps2  OutDataTypeStr=boolean
      settings: AttributesFormatString=|
      | %<relop>
      | %<const>
  Compare To Constant1 : simulink/Logic and Bit Operations/Compare To Constant  relop=>=  const=Flight_Logic.Ax_launch_timer_threshold_sec  OutDataTypeStr=boolean
      settings: AttributesFormatString=|
      | %<relop>
      | %<const>
  Constant : Constant  Value=0
  Enable_Timer_Logic : Subsystem
  Latch_Signal : Subsystem
  Memory : Memory  InheritSampleTime=on  LinearizeAsDelay=on
  Switch : Switch  Criteria=u2 ~= 0
  launch_log : Outport
  TOF_sec : Outport  Port=2
  wires:
  Compare To Constant/1 -> AND/1, Enable_Timer_Logic/1(accel_threshold_log)  "launch_Ax_log"
  Enable_Timer_Logic/1(time_since_launch) -> Switch/1, Compare To Constant1/1
  Compare To Constant1/1 -> AND/2  "launch_timer_log"
  AND/1 -> Latch_Signal/1(signal)
  IMU_Ax_mps2/1 -> Compare To Constant/1
  Latch_Signal/1(signal_latched) -> [launch_latched], launch_log/1  "launch_log"
  [launch_latched] -> Memory/1
  Memory/1 -> Enable_Timer_Logic/2(launch_latched)
  [launch_latched] -> Switch/2
  Switch/1 -> TOF_sec/1  "TOF_sec"
  Constant/1 -> Switch/3

== system Copy_of_Corneto_flight_program_control/Subsystem/PixBlock2/Emulated Pixhawk/Flight_Logic/MECO_Detection_Logic ==
  launch_log : Inport
  IMU_Ax_mps2 : Inport  Port=2
  TOF_sec : Inport  Port=3
  AND : Logic  AllPortsSameDT=off  OutDataTypeStr=boolean
  AND1 : Logic  Operator=OR  AllPortsSameDT=off  OutDataTypeStr=boolean
  Compare To Constant1 : simulink/Logic and Bit Operations/Compare To Constant  relop=>=  const=Flight_Logic.Ax_MECO_timer_threshold_sec  OutDataTypeStr=boolean
      settings: AttributesFormatString=|
      | %<relop>
      | %<const>
  Compare To Constant2 : simulink/Logic and Bit Operations/Compare To Constant  relop=<=  const=0  OutDataTypeStr=boolean
      settings: AttributesFormatString=|
      | %<relop>
      | %<const>
  Compare To Constant3 : simulink/Logic and Bit Operations/Compare To Constant  relop=>=  const=Flight_Logic.MECO_timeout_TOF_sec  OutDataTypeStr=boolean
      settings: AttributesFormatString=|
      | %<relop>
      | %<const>
  Enable_Timer_Logic : Subsystem
  Latch_Signal : Subsystem
  MECO_log : Outport
  wires:
  launch_log/1 -> AND/1
  IMU_Ax_mps2/1 -> Compare To Constant2/1
  Enable_Timer_Logic/1(timer) -> Compare To Constant1/1
  Compare To Constant1/1 -> Latch_Signal/1(signal)  "MECO_timer_log"
  AND/1 -> Enable_Timer_Logic/1(enable_timer)
  AND1/1 -> MECO_log/1  "MECO_log"
  Compare To Constant2/1 -> AND/2  "MECO_Ax_log"
  Latch_Signal/1(signal_latched) -> AND1/1  "MECO_latched"
  TOF_sec/1 -> Compare To Constant3/1
  Compare To Constant3/1 -> AND1/2  "MECO_timeout_log"

== system Copy_of_Corneto_flight_program_control/Subsystem/PixBlock2/Emulated Pixhawk/Flight_Logic/Recovery_Logic ==
  apogee_log : Inport
  TOF_sec : Inport  Port=2
  h_m : Inport  Port=3
  AND1 : Logic  Operator=OR  AllPortsSameDT=off  OutDataTypeStr=boolean
  AND2 : Logic  AllPortsSameDT=off  OutDataTypeStr=boolean
  Compare To Constant1 : simulink/Logic and Bit Operations/Compare To Constant  relop=>=  const=Flight_Logic.apogee_recovery_timer_threshold_sec  OutDataTypeStr=boolean
      settings: AttributesFormatString=|
      | %<relop>
      | %<const>
  Compare To Constant3 : simulink/Logic and Bit Operations/Compare To Constant  relop=>=  const=Flight_Logic.recovery_timeout_TOF_sec  OutDataTypeStr=boolean
      settings: AttributesFormatString=|
      | %<relop>
      | %<const>
  Constant : Constant  Value=Flight_Logic.disable_recovery_manual
      settings: AttributesFormatString=%<Value>
  Enable_Timer_Logic : Subsystem
  Latch_Signal : Subsystem
  NOT : Logic  Operator=NOT  AllPortsSameDT=off  OutDataTypeStr=boolean
  Terminator : Terminator
  recovery_log : Outport
  wires:
  Compare To Constant3/1 -> AND1/2  "recovery_timeout_log"
  TOF_sec/1 -> Compare To Constant3/1
  Latch_Signal/1(signal_latched) -> AND1/1  "recovery_latched"
  AND1/1 -> AND2/1
  apogee_log/1 -> Enable_Timer_Logic/1(enable_timer)
  Compare To Constant1/1 -> Latch_Signal/1(signal)  "apogee_recovery_timer_log"
  Enable_Timer_Logic/1(timer) -> Compare To Constant1/1
  h_m/1 -> Terminator/1
  AND2/1 -> recovery_log/1  "recovery_log"
  Constant/1 -> NOT/1  "disable_recovery_manual"
  NOT/1 -> AND2/2

== system Copy_of_Corneto_flight_program_control/Subsystem/PixBlock2/Emulated Pixhawk/Autopilot/Phi_Control/Gain_Lookup ==
  V_mps : Inport
  h_m : Inport  Port=2
  1-D Lookup Table1 : Lookup_n-D  BreakpointsForDimension1=Autopilot.Ay.h_bkpts_m  BreakpointsForDimension2=Autopilot.Ay.V_bkpts_mps  Table=Autopilot.Ay.Kp_r_vec  ExtrapMethod=Clip  UseLastTableValue=on  InternalRulePriority=Speed  RndMeth=Simplest  InputSameDT=on
      settings: InputPortMap=u0,u1
      settings: AttributesFormatString=|
      | %<Table>
      | %<BreakpointsForDimension1>
      | %<BreakpointsForDimension2>
  1-D Lookup Table2 : Lookup_n-D  BreakpointsForDimension1=Autopilot.Ay.h_bkpts_m  BreakpointsForDimension2=Autopilot.Ay.V_bkpts_mps  Table=Autopilot.Ay.Kp_ay_vec  ExtrapMethod=Clip  UseLastTableValue=on  InternalRulePriority=Speed  RndMeth=Simplest  InputSameDT=on
      settings: InputPortMap=u0,u1
      settings: AttributesFormatString=|
      | %<Table>
      | %<BreakpointsForDimension1>
      | %<BreakpointsForDimension2>
  1-D Lookup Table3 : Lookup_n-D  BreakpointsForDimension1=Autopilot.Phi.h_bkpts_m  BreakpointsForDimension2=Autopilot.Phi.V_bkpts_mps  Table=Autopilot.Phi.Kp_p_vec  ExtrapMethod=Clip  UseLastTableValue=on  InternalRulePriority=Speed  RndMeth=Simplest  InputSameDT=on
      settings: InputPortMap=u0,u1
      settings: AttributesFormatString=|
      | %<Table>
      | %<BreakpointsForDimension1>
      | %<BreakpointsForDimension2>
  1-D Lookup Table4 : Lookup_n-D  BreakpointsForDimension1=Autopilot.Phi.h_bkpts_m  BreakpointsForDimension2=Autopilot.Phi.V_bkpts_mps  Table=Autopilot.Phi.Ki_phi_vec  ExtrapMethod=Clip  UseLastTableValue=on  InternalRulePriority=Speed  RndMeth=Simplest  InputSameDT=on
      settings: InputPortMap=u0,u1
      settings: AttributesFormatString=|
      | %<Table>
      | %<BreakpointsForDimension1>
      | %<BreakpointsForDimension2>
  1-D Lookup Table5 : Lookup_n-D  BreakpointsForDimension1=Autopilot.Phi.h_bkpts_m  BreakpointsForDimension2=Autopilot.Phi.V_bkpts_mps  Table=Autopilot.Phi.Kp_phi_vec  ExtrapMethod=Clip  UseLastTableValue=on  InternalRulePriority=Speed  RndMeth=Simplest  InputSameDT=on
      settings: InputPortMap=u0,u1
      settings: AttributesFormatString=|
      | %<Table>
      | %<BreakpointsForDimension1>
      | %<BreakpointsForDimension2>
  1-D Lookup Table6 : Lookup_n-D  BreakpointsForDimension1=Autopilot.Ay.h_bkpts_m  BreakpointsForDimension2=Autopilot.Ay.V_bkpts_mps  Table=Autopilot.Ay.Ki_ay_vec  ExtrapMethod=Clip  UseLastTableValue=on  InternalRulePriority=Speed  RndMeth=Simplest  InputSameDT=on
      settings: InputPortMap=u0,u1
      settings: AttributesFormatString=|
      | %<Table>
      | %<BreakpointsForDimension1>
      | %<BreakpointsForDimension2>
  Bus Creator1 : BusCreator  Inputs=6
  V_mps D{1..5} (5 alike) : InportShadow
  h_m D{1..5} (5 alike) : InportShadow  Port=2
  Gains : Outport
  wires:
  h_m/1 -> 1-D Lookup Table3/1
  Bus Creator1/1 -> Gains/1
  1-D Lookup Table5/1 -> Bus Creator1/3  "Kp_phi"
  1-D Lookup Table4/1 -> Bus Creator1/2  "Ki_phi"
  1-D Lookup Table3/1 -> Bus Creator1/1  "Kp_p"
  V_mps/1 -> 1-D Lookup Table3/2
  h_m D1/1 -> 1-D Lookup Table4/1
  V_mps D1/1 -> 1-D Lookup Table4/2
  h_m D2/1 -> 1-D Lookup Table5/1
  V_mps D2/1 -> 1-D Lookup Table5/2
  1-D Lookup Table2/1 -> Bus Creator1/6  "Kp_ay"
  1-D Lookup Table6/1 -> Bus Creator1/5  "Ki_ay"
  1-D Lookup Table1/1 -> Bus Creator1/4  "Kp_r"
  h_m D3/1 -> 1-D Lookup Table1/1
  V_mps D3/1 -> 1-D Lookup Table1/2
  h_m D4/1 -> 1-D Lookup Table6/1
  V_mps D4/1 -> 1-D Lookup Table6/2
  h_m D5/1 -> 1-D Lookup Table2/1
  V_mps D5/1 -> 1-D Lookup Table2/2

== system Copy_of_Corneto_flight_program_control/Subsystem/PixBlock2/Emulated Pixhawk/Flight_Logic/Apogee_Detection_Logic/Enable_Timer_Logic ==
  enable_timer : Inport
  Constant : Constant
  Constant1 : Constant  Value=0
  Discrete-Time Integrator : DiscreteIntegrator  ExternalReset=level  InitialConditionSource=external  SampleTime=-1  ICPrevOutput=DiscIntNeverNeededParam  ICPrevScaledInput=DiscIntNeverNeededParam
  NOT : Logic  Operator=NOT  AllPortsSameDT=off  OutDataTypeStr=boolean
  timer : Outport
  wires:
  NOT/1 -> Discrete-Time Integrator/2
  Discrete-Time Integrator/1 -> timer/1  "apogee_detect_timer_sec"
  Constant1/1 -> Discrete-Time Integrator/3
  Constant/1 -> Discrete-Time Integrator/1
  enable_timer/1 -> NOT/1  "enable_timer"

== system Copy_of_Corneto_flight_program_control/Subsystem/PixBlock2/Emulated Pixhawk/Flight_Logic/Apogee_Detection_Logic/Latch_Signal ==
  signal : Inport
  Memory : Memory  InheritSampleTime=on
  Switch1 : Switch  Criteria=u2 ~= 0
      settings: AttributesFormatString=%<Criteria>
  signal_latched : Outport
  wires:
  signal/1 -> Switch1/2, Switch1/1
  Switch1/1 -> Memory/1, signal_latched/1
  Memory/1 -> Switch1/3

== system Copy_of_Corneto_flight_program_control/Subsystem/PixBlock2/Emulated Pixhawk/Flight_Logic/Launch_Detection_Logic/Enable_Timer_Logic ==
  accel_threshold_log : Inport
  launch_latched : Inport  Port=2
  AND : Logic  Operator=OR  AllPortsSameDT=off  OutDataTypeStr=boolean
  Constant : Constant
  Constant1 : Constant  Value=0
  Discrete-Time Integrator : DiscreteIntegrator  ExternalReset=level  InitialConditionSource=external  SampleTime=-1  ICPrevOutput=DiscIntNeverNeededParam  ICPrevScaledInput=DiscIntNeverNeededParam
  NOT : Logic  Operator=NOT  AllPortsSameDT=off  OutDataTypeStr=boolean
  time_since_launch : Outport
  wires:
  launch_latched/1 -> AND/2
  AND/1 -> NOT/1  "enable_timer"
  Constant/1 -> Discrete-Time Integrator/1
  Constant1/1 -> Discrete-Time Integrator/3
  Discrete-Time Integrator/1 -> time_since_launch/1  "launch_detect_timer_sec"
  accel_threshold_log/1 -> AND/1
  NOT/1 -> Discrete-Time Integrator/2

== system Copy_of_Corneto_flight_program_control/Subsystem/PixBlock2/Emulated Pixhawk/Flight_Logic/Launch_Detection_Logic/Latch_Signal ==
  signal : Inport
  Memory : Memory  InheritSampleTime=on  LinearizeAsDelay=on
  Switch1 : Switch  Criteria=u2 ~= 0
      settings: AttributesFormatString=%<Criteria>
  signal_latched : Outport
  wires:
  Memory/1 -> Switch1/3
  Switch1/1 -> signal_latched/1, Memory/1
  signal/1 -> Switch1/1, Switch1/2

== system Copy_of_Corneto_flight_program_control/Subsystem/PixBlock2/Emulated Pixhawk/Flight_Logic/MECO_Detection_Logic/Enable_Timer_Logic ==
  enable_timer : Inport
  Constant : Constant
  Constant1 : Constant  Value=0
  Discrete-Time Integrator : DiscreteIntegrator  ExternalReset=level  InitialConditionSource=external  SampleTime=-1  ICPrevOutput=DiscIntNeverNeededParam  ICPrevScaledInput=DiscIntNeverNeededParam
  NOT : Logic  Operator=NOT  AllPortsSameDT=off  OutDataTypeStr=boolean
  timer : Outport
  wires:
  enable_timer/1 -> NOT/1  "enable_timer"
  Constant/1 -> Discrete-Time Integrator/1
  Constant1/1 -> Discrete-Time Integrator/3
  Discrete-Time Integrator/1 -> timer/1  "MECO_detect_timer_sec"
  NOT/1 -> Discrete-Time Integrator/2

== system Copy_of_Corneto_flight_program_control/Subsystem/PixBlock2/Emulated Pixhawk/Flight_Logic/MECO_Detection_Logic/Latch_Signal ==
  signal : Inport
  Memory : Memory  InheritSampleTime=on
  Switch1 : Switch  Criteria=u2 ~= 0
      settings: AttributesFormatString=%<Criteria>
  signal_latched : Outport
  wires:
  Memory/1 -> Switch1/3
  Switch1/1 -> signal_latched/1, Memory/1
  signal/1 -> Switch1/1, Switch1/2

== system Copy_of_Corneto_flight_program_control/Subsystem/PixBlock2/Emulated Pixhawk/Flight_Logic/Recovery_Logic/Enable_Timer_Logic ==
  enable_timer : Inport
  Constant : Constant
  Constant1 : Constant  Value=0
  Discrete-Time Integrator : DiscreteIntegrator  ExternalReset=level  InitialConditionSource=external  SampleTime=-1  ICPrevOutput=DiscIntNeverNeededParam  ICPrevScaledInput=DiscIntNeverNeededParam
  NOT : Logic  Operator=NOT  AllPortsSameDT=off  OutDataTypeStr=boolean
  timer : Outport
  wires:
  NOT/1 -> Discrete-Time Integrator/2
  Discrete-Time Integrator/1 -> timer/1  "recovery_detect_timer_sec"
  Constant1/1 -> Discrete-Time Integrator/3
  Constant/1 -> Discrete-Time Integrator/1
  enable_timer/1 -> NOT/1  "enable_timer"

== system Copy_of_Corneto_flight_program_control/Subsystem/PixBlock2/Emulated Pixhawk/Flight_Logic/Recovery_Logic/Latch_Signal ==
  signal : Inport
  Memory : Memory  InheritSampleTime=on
  Switch1 : Switch  Criteria=u2 ~= 0
      settings: AttributesFormatString=%<Criteria>
  signal_latched : Outport
  wires:
  signal/1 -> Switch1/2, Switch1/1
  Switch1/1 -> Memory/1, signal_latched/1
  Memory/1 -> Switch1/3

== matlab function Copy_of_Corneto_flight_program_control/MATLAB Function ==
  data: vx input; y output; vy input; vz input
function y = fcn(vx,vy,vz)

y = double(norm([vx vy vz]));
end

== matlab function Copy_of_Corneto_flight_program_control/Subsystem/MATLAB Function ==
  data: vx input; y output; vy input; vz input
function y = fcn(vx,vy,vz)

y = double(norm([vx vy vz]));
end
